simulink model "psb3phsignalseq"  (Simulink 6.0)
settings: Solver=ode23tb  SolverMode=SingleTasking  StartTime=0.0  StopTime=0.2  MaxStep=5e-5  RelTol=1e-3  AbsTol=1e-2
InitFcn:
  | powericon('psbinitsys',bdroot);
libraries: powerlib2 x6, powerlib_extras x2
settings Model: Creator=sybille  LastModifiedBy=batserve  ExtModeTrigMode=oneshot  ExtModeArmWhenConnect=off  ExtModeAutoUpdateStatusClock=off  ProdHWDeviceType=Specified
settings DataIOCC: Decimation=10  LimitDataPoints=off  SaveFinalState=on  SaveOutput=off  SignalLoggingName=sigsOut
settings OptimizationCC: BlockReduction=off  BooleanDataType=off
settings DebuggingCC: CheckExecutionContextPreStartOutputMsg=on  CheckExecutionContextRuntimeOutputMsg=on  SolverPrmCheckMsg=none  UnconnectedInputMsg=none  UnconnectedOutputMsg=none
settings HardwareCC: ProdBitPerShort=32  ProdBitPerInt=16  ProdHWDeviceType=Specified  TargetUnknown=on
settings RTWCC: TemplateMakefile=grt_vc.tmf

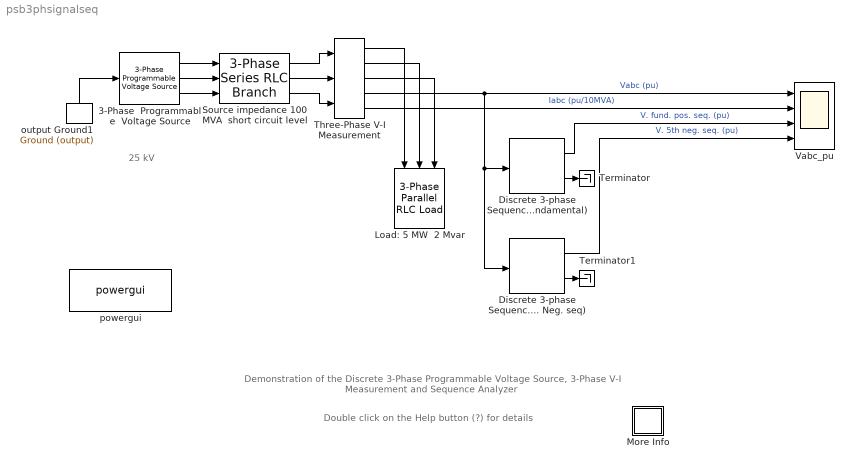
== system psb3phsignalseq ==
  note: Demonstration of the Discrete 3-Phase Programmable Voltage Source,
      |  3-Phase V-I Measurement and Sequence Analyzer
  note: Double click on the Help button (?) for details
  note: 25 kV
  3-Phase  Programmable  Voltage Source : powerlib2/Electrical Sources/3-Phase  Programmable  Voltage Source  Par_Vps_LLrms="[25e3 0  60]"  VariationEntity=Amplitude  VariationType=Step  VariationStep=0.5  VariationRate=10  VariationMag=0.3  VariationFreq=2  Par_Timing_Variation=[0.05 1]  SinglePhase=off  Yampli=[1 0.8 1.2 1.0]  Xtime=[0 0.1 0.15 0.2]  HarmonicGeneration=on  Par_HarmoA_pu=[5 0.08 -45 0]  Par_HarmoB_pu=[2 0 0 2]  Par_Timing_Harmo="[0.1  1]"
  Discrete 3-phase Sequence Analyzer (5th harm. Neg. seq) : powerlib_extras/Discrete Measurements/Discrete 3-phase Sequence Analyzer  Freq=60  n=5  seq=Negative  Par_Init=[0 0]  Ts=50e-6
  Discrete 3-phase Sequence Analyzer (Fundamental) : powerlib_extras/Discrete Measurements/Discrete 3-phase Sequence Analyzer  Freq=60  n=1  seq=Positive  Par_Init=[0 0]  Ts=50e-6
  Load: 5 MW  2 Mvar : powerlib2/Elements/3-Phase Parallel RLC Load  Orientation=down  Vpp=25e3  fn=60  P3=5e6  QL3=0  QC3=2e6
  More Info : Subsystem
      mask Display: disp('?')
  Source impedance 100 MVA  short circuit level : powerlib2/Elements/3-Phase Series RLC Branch   R=25^2/100/10  L=25^2/100/377  C=inf
  Terminator : Terminator
  Terminator1 : Terminator
  Three-Phase V-I Measurement : powerlib2/Measurements/Three-Phase V-I Measurement  Tag=PoWeRsYsTeMmEaSuReMeNt  VChoice=phase-to-ground  ualv=off  labelV=V1  Vpu=on  Vbase=25e3  IChoice=yes  ualc=off  labelC=I1  Ppu=on  Pbase=10e6  OutputType=Magnitude  PhasorSimulation=off  PSBequivalent=1  PSBOutputType=11100
  Vabc_pu : Scope  NumInputPorts=4
      settings: TimeRange=0.2  YMin=-2~-2~0~0  YMax=2~1~2~0.2  DataFormat=Array  SampleInput=on
  output Ground1 : powerlib2/Connectors/Ground (output)  Tag=PoWeRsYsTeMbLoCk  Orientation=up  PSBOutputType=1
  powergui : powerlib2/powergui  Frange=[0:2:500]  Ylog=off  Xlog=off  save=off  variable=ZData  ZoomFFT=on  StartTime=0.0  cycles=1  DisplayStyle=off  fundamental=60  FreqAxis=off  MaxFrequency=1000  frequencyindice=1  frequencyindicesteady=1  RmsSteady=1  display=off  Ts=50e-6  methode=off  frequency=60  echomessages=off
  wires:
  Source impedance 100 MVA  short circuit level/1 -> Three-Phase V-I Measurement/1
  Source impedance 100 MVA  short circuit level/2 -> Three-Phase V-I Measurement/2
  Source impedance 100 MVA  short circuit level/3 -> Three-Phase V-I Measurement/3
  Discrete 3-phase Sequence Analyzer (Fundamental)/1 -> Vabc_pu/3  "V. fund. pos. seq. (pu)"
  Discrete 3-phase Sequence Analyzer (5th harm. Neg. seq)/1 -> Vabc_pu/4  "V. 5th neg. seq. (pu)"
  Three-Phase V-I Measurement/1 -> Load: 5 MW  2 Mvar/1
  Three-Phase V-I Measurement/2 -> Load: 5 MW  2 Mvar/2
  Three-Phase V-I Measurement/3 -> Load: 5 MW  2 Mvar/3
  Three-Phase V-I Measurement/5 -> Vabc_pu/2  "Iabc (pu/10MVA)"
  Three-Phase V-I Measurement/4 -> Vabc_pu/1, Discrete 3-phase Sequence Analyzer (Fundamental)/1, Discrete 3-phase Sequence Analyzer (5th harm. Neg. seq)/1  "Vabc (pu)"
  Discrete 3-phase Sequence Analyzer (Fundamental)/2 -> Terminator/1
  Discrete 3-phase Sequence Analyzer (5th harm. Neg. seq)/2 -> Terminator1/1
  3-Phase  Programmable  Voltage Source/1 -> Source impedance 100 MVA  short circuit level/1
  3-Phase  Programmable  Voltage Source/2 -> Source impedance 100 MVA  short circuit level/2
  3-Phase  Programmable  Voltage Source/3 -> Source impedance 100 MVA  short circuit level/3
  output Ground1/1 -> 3-Phase  Programmable  Voltage Source/1

== system psb3phsignalseq/More Info ==
  note: Circuit Description
  note: This demonstration ilustrates use of the 3-Phase Programmable Voltage Source,
      | 3-Phase V-I Measurement, and Sequence Analyzer blocks
  note: A  25kV, 100 MVA short-circuit level,  equivalent network feeds a 5MW, 2 Mvar capacitive load.
      |
      | The internal voltage of the source is controlled by the Discrete 3-phase Programmable Voltage Source block.
      |
      | Open the source dialog box and look at the parameters controlling the voltage. A positive-sequence of
      | 1.0 pu, 0 degrees is specified. At t = 0.05 s a step of 0.5 pu is applied on positive-sequence voltage magnitude,
      | then, at t = 0.1 s, 0.08 pu of 5th harmonic in negative sequence is added on the 1.5 pu voltage.
      |
      | In order to start simulation in steady state, the three voltage sources are initialized  with a
      | positive-sequence voltage of 25 kV, 0 degree, 60 Hz.
      |
      | The Three-Phase V-I Measurement block allows to monitor the three load voltages and currents.
      | Open its dialog box and see how this block allows to output the voltages and currents in pu.
      |
      | Two Discrete 3-phase Sequence Analyzer blocks are used to monitor the positive-sequeence of the three fundamental voltages Va, Vb, Vc
      | and the negative-sequence component of the 5th harmonic.
      |
      | The whole system, (power network, programmable source and sequence analyzers) is discretized at a 50 us sample time.
  note: Demonstration
  note: Choose  Simulation/Start and observe the  voltage and current waveforms.
      |
      | The simulation starts in steady state with 1 pu voltage.
      | At t = 0.05 sec the internal voltage is increased to 1.5 pu. At t = 0.10 sec. 0.08 pu of 5th harmonic internal voltage is added.
      |
      | Observe the fundamental component (pos. seq.) and the 5th harmonic component  (neg. seq.) measured by the two sequence analyzers.
      | The 0.08 pu 5th harmonic internal voltage is amplified at 0.14 pu at the load terminals
      | As the sequence analyzers use Fourier analysis, their response time is one cycle.
  note: G. Sybille (Hydro-Quebec)
